simulink subsystem "triggered_sub_test"  (R2022b)
settings: Solver=VariableStepAuto  StartTime=0.0  StopTime=10.0  RelTol=1e-3
settings Model: Creator=User  LastModifiedBy=User

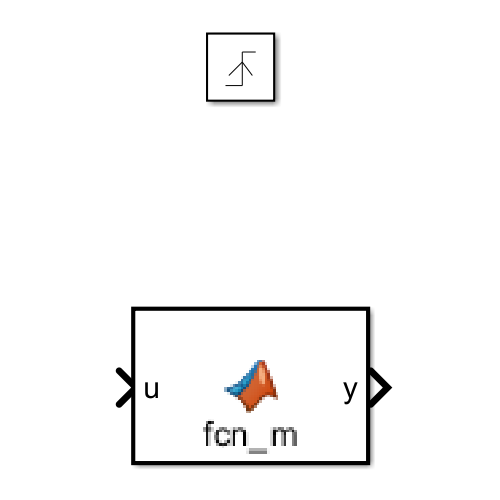
[thumbnail: Simulink's stored preview of the top-level diagram]
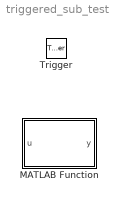
== system triggered_sub_test ==
  Trigger : TriggerPort  VariantControl=(inherit)  PortDimensions=1
  MATLAB Function : MATLAB Function  TreatAsAtomicUnit=on

== matlab function triggered_sub_test/MATLAB Function ==
  data: u input; y output
function y = fcn_m(u)
    y = fcn(u);
    
end
